simulink model "PMSM_SMO"  (R2023a)
settings: Solver=ode3  StartTime=0.0  StopTime=0.15  FixedStep=2e-7  RelTol=1e-4  EnableMultiTasking=on
InitFcn:
  | R = 0.2875;
  | Ld = 0.002;
  | Lq = 0.004;
  | M=0.4;
  | K=0.2;
values from neighbouring files (symbols this model uses):
  A = [Ld/r Lq/r]    [Motor_PIParam_Get2.m]
  flux = 2.5    [Copy_of_imitate_MPTA_MPTV.m]    (also in Motor_PIParam_Get2.m = 0.646; imitate_MPTA_MPTV.m)
undefined symbols (not defined in the file or in its folder): L
libraries: spsDCVoltageSourceLib x1, spsGroundLib x1, spsPermanentMagnetSynchronousMachineLib x1, simulink x1, spsThreePhaseVIMeasurementLib x1, spsUniversalBridgeLib x1, spspowerguiLib x1
settings Model: Creator=Lei  LastModifiedBy=yll
settings SolverCC: AlgebraicLoopSolver=TrustRegion
settings DataIOCC: LimitDataPoints=on  SaveFormat=Array  SignalLoggingSaveFormat=ModelDataLogs  ReturnWorkspaceOutputs=off
settings OptimizationCC: ExpressionDepthLimit=2147483647  InitFltsAndDblsToZero=on  LifeSpan=inf
settings DebuggingCC: SaveWithParameterizedLinksMsg=none  UnderspecifiedInitializationDetection=Classic  MergeDetectMultiDrivingBlocksExec=none  SignalResolutionControl=TryResolveAllWithWarning  SolverPrmCheckMsg=warning  MultiTaskDSMMsg=warning  MultiTaskCondExecSysMsg=none  FcnCallInpInsideContextMsg=warning  UnconnectedInputMsg=warning  UnconnectedOutputMsg=warning  StateNameClashWarn=warning  SFUnexpectedBacktrackingDiag=warning  SFNoUnconditionalDefaultTransitionDiag=warning  SFExecutionAtInitializationDiag=none  ArithmeticOperatorsInVariantConditions=warning
settings HardwareCC: ProdBitPerPointer=32  ProdBitPerSizeT=32  ProdBitPerPtrDiffT=32  ProdLargestAtomicFloat=None  ProdIntDivRoundTo=Undefined  ProdEndianess=Unspecified  ProdWordSize=32  ProdHWDeviceType=32-bit Generic
settings ModelReferenceCC: PropagateSignalLabelsOutOfModel=off
settings SFSimCC: SimUseLocalCustomCode=off  CustomCodeUndefinedFunction=UseInterfaceOnly
settings RTWCC: RTWUseLocalCustomCode=off
settings CodeAppCC: StateflowObjectComments=on
settings GRTTargetCC: TargetFcnLib=ansi_tfl_tmw.mat  TargetLangStandard=C89/C90 (ANSI)  CombineOutputUpdateFcns=off  GRTInterface=on
settings ConfigComp: CovMetricSettings=dw  CovSaveCumulativeToWorkspaceVar=on  CovSaveSingleToWorkspaceVar=on  CovExternalEMLEnable=off  CovSFcnEnable=off
settings SimscapeCC: SimscapeNormalizeSystem=off

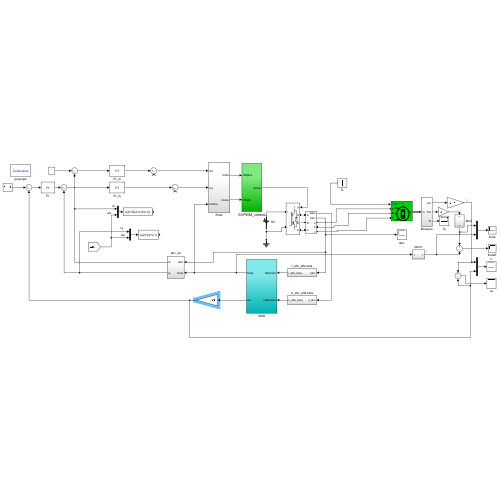
[thumbnail: Simulink's stored preview of the top-level diagram]
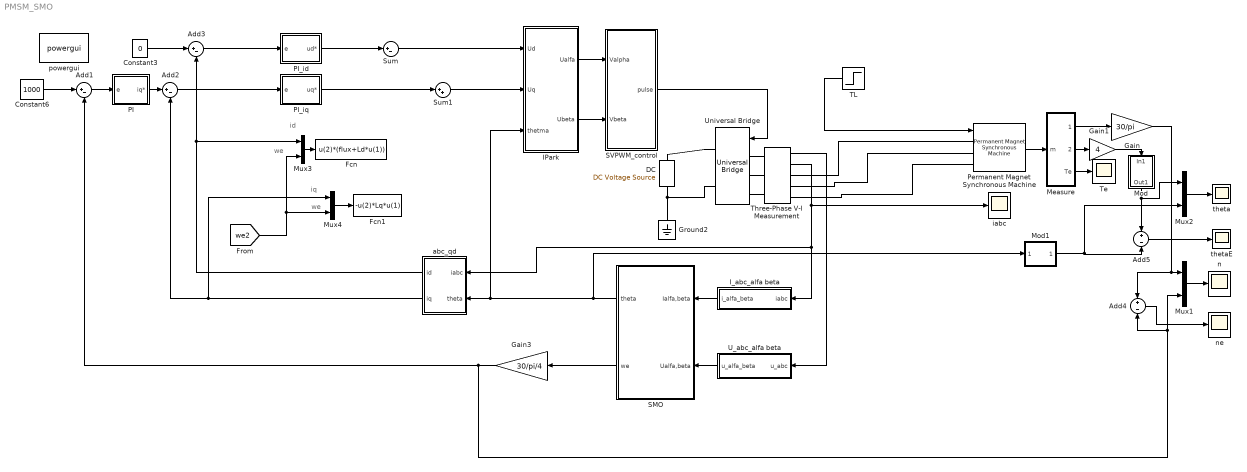
== system PMSM_SMO ==
  note: id
  note: we
  note: iq
  note: we
  Add1 : Sum  Inputs=|+-
  Add2 : Sum  Inputs=|+-
  Add3 : Sum  Inputs=|+-
  Add4 : Sum  Inputs=+|-
  Add5 : Sum  Inputs=+|-
  Constant3 : Constant  Value=0
  Constant6 : Constant  Value=1000
  "DC " : spsDCVoltageSourceLib/DC Voltage Source  Amplitude=311  Measurements=None
  Fcn : Fcn  Expr=u(2)*(flux+Ld*u(1))
  Fcn1 : Fcn  Expr=-u(2)*Lq*u(1)
  Gain : Gain  Gain=30/pi
  Gain1 : Gain  Gain=4
  Gain3 : Gain  Gain=30/pi/4
  Ground2 : spsGroundLib/Ground  LConnTagsString=a
  IPark : Subsystem
  I_abc_alfa beta : Subsystem
  Measure : Subsystem
  Mod : Subsystem
  Mod1 : Subsystem
  Mux{1..4} (4 alike) : Mux  Inputs=2
  PI : Subsystem
      mask Display: disp('PI')
  PI_id : Subsystem
      mask Display: disp('PI')
  PI_iq : Subsystem
      mask Display: disp('PI')
  Permanent Magnet Synchronous Machine : spsPermanentMagnetSynchronousMachineLib/Permanent Magnet Synchronous Machine  NbPhases=3  FluxDistribution=Sinusoidal  RotorType=Salient-pole  MechanicalLoad=Torque Tm  PresetModel=No  ShowDetailedParameters=on  MeasurementBus=off  Resistance=2.8750  Inductance=8.5e-3  dqInductances=[Ld, Lq]  La=0.000835  MachineConstant=Flux linkage established by magnets (V.s)  Flux=0.175  VoltageCst=126.966  TorqueCst=1.05  Flat=120  Mechanical="[ 1e-3, 0,  4 ]"  PolePairs=4  InitialConditions=[0,0, 0,0]  InitialConditions5ph=[0 0 0 0 0 0]  RefAngle=90 degrees behind phase A axis (modified Park)  IterativeDiscreteModel=Trapezoidal non iterative  TsBlock=-1  TsPowergui=0
  SMO : Subsystem
  SVPWM_control : Subsystem
  Sum : Sum  Inputs=|+-
  Sum1 : Sum  Inputs=|++
  TL : Step  Time=0.1  After=0  SampleTime=0
  Te : Scope
  Three-Phase V-I Measurement : spsThreePhaseVIMeasurementLib/Three-Phase V-I Measurement  VoltageMeasurement=phase-to-ground  SetLabelV=off  LabelV=Vabc  Vpu=off  VpuLL=off  CurrentMeasurement=yes  SetLabelI=off  LabelI=Iabc  Ipu=off  Pbase=100e6  Vbase=500e3  OutputType=Complex  PhasorSimulation=off  PSBequivalent=0
  U_abc_alfa beta : Subsystem
  Universal Bridge : spsUniversalBridgeLib/Universal Bridge  Arms=3  SnubberResistance=1e5  SnubberCapacitance=inf  Device=IGBT / Diodes  Ron=1e-3  Lon=0  ForwardVoltages="[  0  0  ]"  ForwardVoltage=0  GTOparameters=[ 10e-6 , 20e-6 ]  IGBTparameters=[ 1e-6 , 2e-6 ]  Measurements=None  Measurements_2=None  converterType=Rectifier
  abc_qd : Subsystem
  iabc : Scope
  n : Scope
  ne : Scope
  powergui : spspowerguiLib/powergui  Priority=1  SimulationMode=Continuous  SampleTime=50e-6  frequency=60  Iterations=50  frequencyindice=0  Pbase=100e6  ErrMax=1e-4  UnitsV=kV  UnitsW=MW  buscounter=0  FunctionMessages=off  echomessages=off  EnableUseOfTLC=off  CurrentSourceSwitches=off  DisableSnubberDevices=off  DisableRonSwitches=off  DisableVfSwitches=off  DisplayEquations=off  AutomaticDiscreteSolvers=off  SolverType=Tustin/Backward Euler (TBE)  Interpol=off  ExternalGateDelay=off  methode=off  Ts=100  x0status=blocks  SPID=off  SwTol=0  HookPort=off  NonlinearTolerance=1e-4  nMaxIteration=100  ContinueOnMaxIteration=off  RestoreLinks=warning  ResistiveCurrentMeasurement=off  Frange=[0:2:500]  Ylog=off  Xlog=on  ShowGrid=off  save=off  variable=ZData  structure=0  ZoomFFT=off  StartTime=0.0  cycles=1  DisplayStyle=1  fundamental=60  FreqAxis=off  MaxFrequency=1000  frequencyindicesteady=1  RmsSteady=1  display=off
  theta : Scope
  thetaE : Scope
  wires:
  Constant3/1 -> Add3/1
  Add1/1 -> PI/1(e)
  Constant6/1 -> Add1/1
  SVPWM_control/1(pulse) -> Universal Bridge/1
  IPark/1(Ualfa) -> SVPWM_control/1(Valpha)
  IPark/2(Ubeta) -> SVPWM_control/2(Vbeta)
  TL/1 -> Permanent Magnet Synchronous Machine/1
  PI/1(iq*) -> Add2/1
  Gain3/1 -> Add1/2, Add4/2, Mux1/2
  SMO/2(we) -> Gain3/1
  Permanent Magnet Synchronous Machine/1 -> Measure/1(m)
  Measure/1(wm) -> Gain/1
  Measure/2(The) -> Gain1/1
  Measure/3(Te) -> Te/1
  Three-Phase V-I Measurement/1 -> U_abc_alfa beta/1(u_abc)
  Add2/1 -> PI_iq/1(e)
  Add3/1 -> PI_id/1(e)
  abc_qd/1(id) -> Mux3/1, Add3/2
  I_abc_alfa beta/1(i_alfa_beta) -> SMO/1(Ialfa,beta)
  U_abc_alfa beta/1(u_alfa_beta) -> SMO/2(Ualfa,beta)
  SMO/1(theta) -> IPark/3(thetma), abc_qd/2(theta), Mod1/1(In1)
  Three-Phase V-I Measurement/2 -> abc_qd/1(iabc), I_abc_alfa beta/1(iabc), iabc/1
  Mux1/1 -> n/1
  Gain/1 -> Add4/1, Mux1/1
  Gain1/1 -> Mod/1(In1)
  Mux2/1 -> theta/1
  Add5/1 -> thetaE/1
  Add4/1 -> ne/1
  Mod/1(Out1) -> Mux2/1, Add5/1
  Mod1/1(Out1) -> Add5/2, Mux2/2
  PI_iq/1(uq*) -> Sum1/1
  Sum1/1 -> IPark/2(Uq)
  Sum/1 -> IPark/1(Ud)
  PI_id/1(ud*) -> Sum/1
  Mux4/1 -> Fcn1/1
  Mux3/1 -> Fcn/1
  abc_qd/2(iq) -> Mux4/1, Add2/2
  [we2] -> Mux4/2, Mux3/2
  connections:
  Universal Bridge/RConn1 -- "DC "/RConn1
  "DC "/LConn1 -- Ground2/LConn1 -- Universal Bridge/RConn2
  Universal Bridge/LConn1 -- Three-Phase V-I Measurement/LConn1
  Universal Bridge/LConn2 -- Three-Phase V-I Measurement/LConn2
  Universal Bridge/LConn3 -- Three-Phase V-I Measurement/LConn3
  Three-Phase V-I Measurement/RConn1 -- Permanent Magnet Synchronous Machine/LConn1
  Three-Phase V-I Measurement/RConn2 -- Permanent Magnet Synchronous Machine/LConn2
  Three-Phase V-I Measurement/RConn3 -- Permanent Magnet Synchronous Machine/LConn3

== system PMSM_SMO/IPark ==
  Ud : Inport
  Uq : Inport  Port=2
  thetma : Inport  Port=3
  Fcn : Fcn  Expr=cos(u[3])*u[2]-sin(u[3])*u[1]
  Fcn1 : Fcn  Expr=sin(u[3])*u[2]+cos(u[3])*u[1]
  Mux : Mux  Inputs=3
  Ualfa : Outport
  Ubeta : Outport  Port=2
  wires:
  Uq/1 -> Mux/1
  Ud/1 -> Mux/2
  thetma/1 -> Mux/3
  Mux/1 -> Fcn/1, Fcn1/1
  Fcn/1 -> Ualfa/1
  Fcn1/1 -> Ubeta/1

== system PMSM_SMO/I_abc_alfa beta ==
  iabc : Inport
  Fcn : Fcn  Expr=(2*u(1)-u(2)-u(3))/3
  Fcn1 : Fcn  Expr=(u(2)-u(3))/(3^(1/2))
  Mux2 : Mux  Inputs=2
  i_alfa_beta : Outport
  wires:
  iabc/1 -> Fcn/1, Fcn1/1
  Mux2/1 -> i_alfa_beta/1
  Fcn/1 -> Mux2/1
  Fcn1/1 -> Mux2/2

== system PMSM_SMO/Measure ==
  m : Inport
  Bus Selector1 : BusSelector  OutputSignals=Rotor speed wm (rad/s),Rotor angle thetam (rad),Electromagnetic torque Te (N*m)
  wm : Outport
  The : Outport  Port=2
  Te : Outport  Port=3
  wires:
  Bus Selector1/2 -> The/1  "<Rotor angle thetam (rad)>"
  Bus Selector1/3 -> Te/1  "<Electromagnetic torque Te (N*m)>"
  m/1 -> Bus Selector1/1
  Bus Selector1/1 -> wm/1  "<Rotor speed wm (rad/s)>"

== system PMSM_SMO/Mod ==
  In1 : Inport
  Constant1 : Constant  Value=pi/4
  Math Function : Math  Operator=mod  SignedPower=on
  Out1 : Outport
  wires:
  Constant1/1 -> Math Function/2
  Math Function/1 -> Out1/1
  In1/1 -> Math Function/1

== system PMSM_SMO/Mod1 ==
  In1 : Inport
  Constant1 : Constant  Value=pi/4
  Math Function : Math  Operator=mod  SignedPower=on
  Out1 : Outport
  wires:
  In1/1 -> Math Function/1
  Math Function/1 -> Out1/1
  Constant1/1 -> Math Function/2

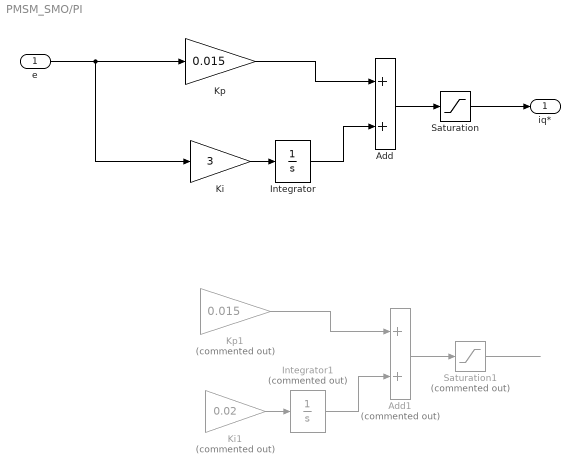
== system PMSM_SMO/PI ==
  e : Inport
  Add : Sum
  Add1 : Sum  Commented=on
  Integrator : Integrator
  Integrator1 : Integrator  Commented=on
  Ki : Gain  Gain=3
  Ki1 : Gain  Commented=on  Gain=0.02
  Kp : Gain  Gain=0.015
  Kp1 : Gain  Commented=on  Gain=0.015
  Saturation : Saturate  UpperLimit=21  LowerLimit=-21
  Saturation1 : Saturate  Commented=on  UpperLimit=21  LowerLimit=-21
  iq* : Outport
  wires:
  Saturation/1 -> iq*/1
  Ki/1 -> Integrator/1
  e/1 -> Kp/1, Ki/1
  Integrator/1 -> Add/2
  Kp/1 -> Add/1
  Add/1 -> Saturation/1
  Kp1/1 -> Add1/1
  Integrator1/1 -> Add1/2
  Ki1/1 -> Integrator1/1
  ? -> Kp1/1, Ki1/1
  Add1/1 -> Saturation1/1
  Saturation1/1 -> ?

== system PMSM_SMO/PI_id ==
  e : Inport
  Add : Sum
  Integrator : Integrator
  Integrator1 : Integrator
  Ki : Gain  Gain=R*2000
  Ki1 : Gain  Gain=R*2000
  Kp : Gain  Gain=20
  Kp1 : Gain  Gain=20
  Saturation : Saturate  UpperLimit=350  LowerLimit=-350
  ud* : Outport
  wires:
  Ki/1 -> Integrator/1
  e/1 -> Kp/1, Ki/1
  Saturation/1 -> ud*/1
  Integrator/1 -> Add/2
  Kp/1 -> Add/1
  Add/1 -> Saturation/1
  Integrator1/1 -> ?
  ? -> Ki1/1
  ? -> Kp1/1
  Kp1/1 -> ?
  Ki1/1 -> Integrator1/1

== system PMSM_SMO/PI_iq ==
  e : Inport
  Add : Sum
  Integrator : Integrator
  Ki : Gain  Gain=R*2000
  Kp : Gain  Gain=20
  Saturation : Saturate  UpperLimit=350  LowerLimit=-350
  uq* : Outport
  wires:
  Ki/1 -> Integrator/1
  e/1 -> Kp/1, Ki/1
  Saturation/1 -> uq*/1
  Integrator/1 -> Add/2
  Kp/1 -> Add/1
  Add/1 -> Saturation/1

== system PMSM_SMO/SMO ==
  Ialfa,beta : Inport
  Ualfa,beta : Inport  Port=2
  Arctan_function1 : Subsystem
  FULL_SMO : Subsystem
  PLL : Subsystem
  SMO : Subsystem
  theta : Outport
  we : Outport  Port=2
  tag scope: we2=global
  wires:
  Arctan_function1/1(theta) -> theta/1
  Arctan_function1/2(we) -> [we2], we/1
  Ualfa,beta/1 -> FULL_SMO/1(Ualfa,beta)
  Ialfa,beta/1 -> FULL_SMO/2(Ialfa,beta)
  FULL_SMO/1(Ealpha^) -> Arctan_function1/1(Ealpha^)
  FULL_SMO/2(Ebeta^) -> Arctan_function1/2(Ebeta)

== system PMSM_SMO/SVPWM_control ==
  Valpha : Inport
  Vbeta : Inport  Port=2
  Repeating Sequence : simulink/Sources/Repeating Sequence  rep_seq_t=[0 0.0001 0.0002]  rep_seq_y=[0 0.0001 0]
  Subsystem : Subsystem
  Subsystem1 : Subsystem
  Subsystem2 : Subsystem
  Subsystem3 : Subsystem
  Subsystem4 : Subsystem
  Subsystem5 : Subsystem
  T : Constant  Value=0.0001
  Vdc : Constant  Value=311
  pulse : Outport
  wires:
  Subsystem5/1(g) -> pulse/1
  Repeating Sequence/1 -> Subsystem5/1(In1)
  Subsystem4/3(Tcm3) -> Subsystem5/4(In4)
  Subsystem4/2(Tcm2) -> Subsystem5/3(In3)
  Subsystem4/1(Tcm1) -> Subsystem5/2(In2)
  Subsystem3/3(Tc) -> Subsystem4/4(In4)
  Subsystem3/2(Tb) -> Subsystem4/3(In3)
  Subsystem3/1(Ta) -> Subsystem4/2(In2)
  Subsystem2/2(T2) -> Subsystem3/3(T2)
  Subsystem2/1(T1) -> Subsystem3/1(T1)
  Subsystem1/3(Z) -> Subsystem2/4(In4)
  Subsystem1/2(Y) -> Subsystem2/3(In3)
  Subsystem1/1(x) -> Subsystem2/2(In2)
  Subsystem/1(N) -> Subsystem4/1(In1), Subsystem2/1(In1)
  Vdc/1 -> Subsystem1/4(Vdc)
  T/1 -> Subsystem3/2(T), Subsystem1/1(T)
  Vbeta/1 -> Subsystem1/2(In2), Subsystem/2(Vbeta)
  Valpha/1 -> Subsystem1/3(In3), Subsystem/1(Valpha)

== system PMSM_SMO/U_abc_alfa beta ==
  u_abc : Inport
  Fcn : Fcn  Expr=(2*u(1)-u(2)-u(3))/3
  Fcn1 : Fcn  Expr=(u(2)-u(3))/(3^(1/2))
  Mux2 : Mux  Inputs=2
  u_alfa_beta : Outport
  wires:
  u_abc/1 -> Fcn/1, Fcn1/1
  Mux2/1 -> u_alfa_beta/1
  Fcn/1 -> Mux2/1
  Fcn1/1 -> Mux2/2

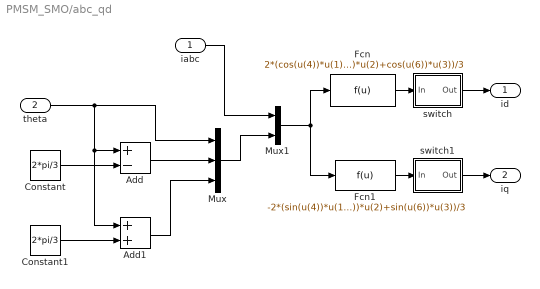
== system PMSM_SMO/abc_qd ==
  iabc : Inport
  theta : Inport  Port=2
  Add : Sum  Inputs=+-
  Add1 : Sum
  Constant : Constant  Value=2*pi/3
  Constant1 : Constant  Value=2*pi/3
  Fcn : Fcn  Expr=2*(cos(u(4))*u(1)+cos(u(5))*u(2)+cos(u(6))*u(3))/3
  Fcn1 : Fcn  Expr=-2*(sin(u(4))*u(1)+sin(u(5))*u(2)+sin(u(6))*u(3))/3
  Mux : Mux  Inputs=3
  Mux1 : Mux  Inputs=2
  switch : Subsystem
  switch1 : Subsystem
  id : Outport
  iq : Outport  Port=2
  wires:
  Constant1/1 -> Add1/2
  Constant/1 -> Add/2
  theta/1 -> Mux/1, Add1/1, Add/1
  Add/1 -> Mux/2
  Add1/1 -> Mux/3
  Mux/1 -> Mux1/2
  iabc/1 -> Mux1/1
  Mux1/1 -> Fcn/1, Fcn1/1
  Fcn/1 -> switch/1(In)
  switch/1(Out) -> id/1
  Fcn1/1 -> switch1/1(In)
  switch1/1(Out) -> iq/1

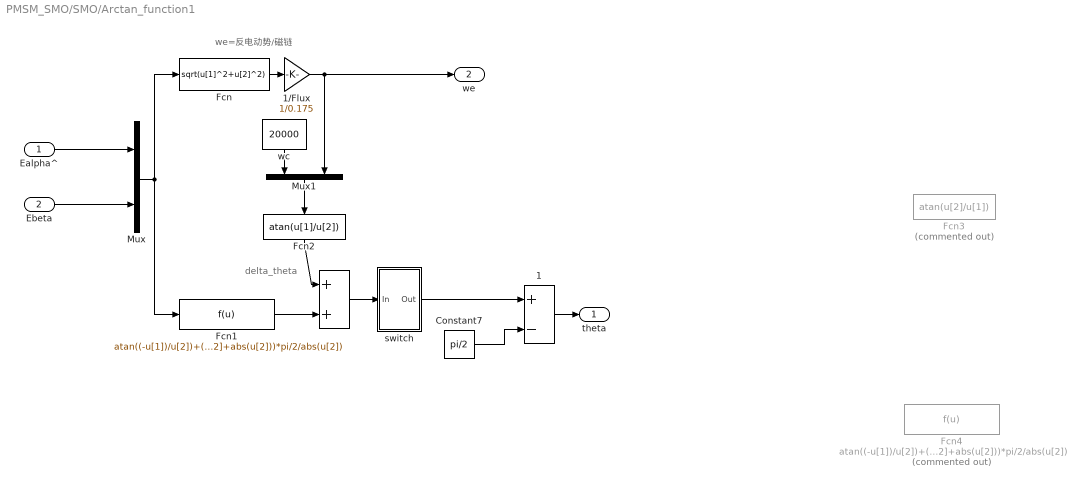
== system PMSM_SMO/SMO/Arctan_function1 ==
  note: we=反电动势/磁链
  note: delta_theta
  Ealpha^ : Inport
  Ebeta : Inport  Port=2
  "  " : Sum
  "  1" : Sum  Inputs=+-
  1/Flux : Gain  Gain=1/0.175
  Constant7 : Constant  Value=pi/2
  Fcn : Fcn  Expr=sqrt(u[1]^2+u[2]^2)
  Fcn1 : Fcn  Expr=atan((-u[1])/u[2])+(-u[2]+abs(u[2]))*pi/2/abs(u[2])
  Fcn2 : Fcn  Expr=atan(u[1]/u[2])
  Fcn3 : Fcn  Commented=on  Expr=atan(u[2]/u[1])
  Fcn4 : Fcn  Commented=on  Expr=atan((-u[1])/u[2])+(-u[2]+abs(u[2]))*pi/2/abs(u[2])
  Mux : Mux  Inputs=2
  Mux1 : Mux  Inputs=2
  switch : Subsystem
  wc : Constant  Value=20000
  theta : Outport
  we : Outport  Port=2
  wires:
  Mux/1 -> Fcn/1, Fcn1/1
  Fcn/1 -> 1/Flux/1
  1/Flux/1 -> we/1, Mux1/2
  Fcn1/1 -> "  "/2
  "  "/1 -> switch/1(In)
  Mux1/1 -> Fcn2/1
  Fcn2/1 -> "  "/1
  wc/1 -> Mux1/1
  switch/1(Out) -> "  1"/1
  Ebeta/1 -> Mux/2
  Ealpha^/1 -> Mux/1
  Constant7/1 -> "  1"/2
  "  1"/1 -> theta/1

== system PMSM_SMO/SMO/FULL_SMO ==
  note: 低通滤波器
  Ualfa,beta : Inport
  Ialfa,beta : Inport  Port=2
  Demux1 : Demux  Outputs=2
  Demux2 : Demux  Outputs=2
  凸极 : Subsystem
  Ealpha^ : Outport
  Ebeta^ : Outport  Port=2
  wires:
  Demux2/2 -> 凸极/4(Ibeta)
  Demux2/1 -> 凸极/3(Ialfa)
  Demux1/2 -> 凸极/2(Ubeta)
  Demux1/1 -> 凸极/1(Ualfa)
  Ualfa,beta/1 -> Demux1/1
  Ialfa,beta/1 -> Demux2/1
  凸极/1(E_alpha_pre) -> Ealpha^/1
  凸极/2(E_beta_pre) -> Ebeta^/1

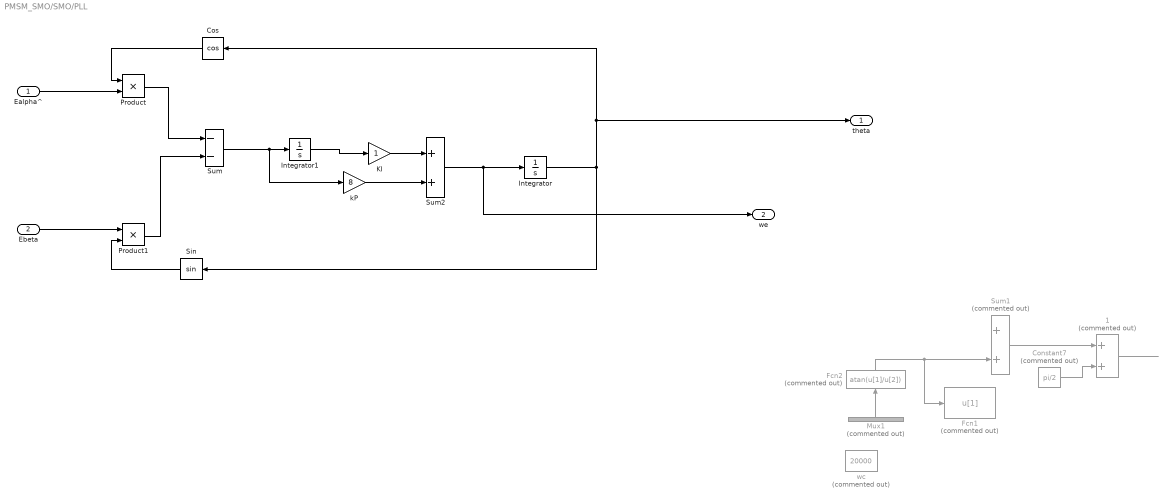
== system PMSM_SMO/SMO/PLL ==
  Ealpha^ : Inport
  Ebeta : Inport  Port=2
  "  1" : Sum  Commented=on
  Constant7 : Constant  Commented=on  Value=pi/2
  Cos : Trigonometry  Operator=cos
  Fcn1 : Fcn  Commented=on  Expr=u[1]
  Fcn2 : Fcn  Commented=on  Expr=atan(u[1]/u[2])
  Integrator : Integrator
  Integrator1 : Integrator
  KI : Gain
  Mux1 : Mux  Commented=on  Inputs=2
  Product : Product
  Product1 : Product
  Sin : Trigonometry
  Sum : Sum  Inputs=--
  Sum1 : Sum  Commented=on
  Sum2 : Sum
  kP : Gain  Gain=8
  wc : Constant  Commented=on  Value=20000
  theta : Outport
  we : Outport  Port=2
  wires:
  Product/1 -> Sum/1
  Product1/1 -> Sum/2
  Cos/1 -> Product/1
  Sin/1 -> Product1/2
  kP/1 -> Sum2/2
  KI/1 -> Sum2/1
  Integrator1/1 -> KI/1
  Sum/1 -> kP/1, Integrator1/1
  Ebeta/1 -> Product1/1
  Ealpha^/1 -> Product/2
  Sum1/1 -> "  1"/1
  Constant7/1 -> "  1"/2
  "  1"/1 -> ?
  Fcn2/1 -> Fcn1/1, Sum1/2
  ? -> Mux1/2
  ? -> Sum1/1
  Mux1/1 -> Fcn2/1
  Sum2/1 -> we/1, Integrator/1
  Integrator/1 -> Cos/1, theta/1, Sin/1

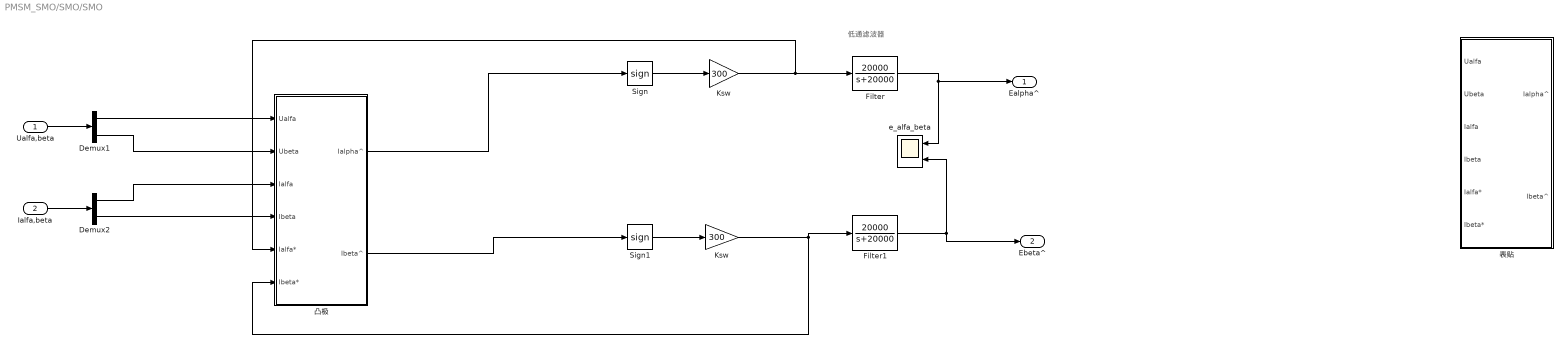
== system PMSM_SMO/SMO/SMO ==
  note: 低通滤波器
  Ualfa,beta : Inport
  Ialfa,beta : Inport  Port=2
  Demux1 : Demux  Outputs=2
  Demux2 : Demux  Outputs=2
  Filter : TransferFcn  Numerator=[20000]  Denominator=[1 20000]
  Filter1 : TransferFcn  Numerator=[20000]  Denominator=[1 20000]
  Ksw : Gain  Gain=300
  "Ksw " : Gain  Gain=300
  Sign : Signum  ZeroCross=off
  Sign1 : Signum  ZeroCross=off
  e_alfa_beta : Scope  NumInputPorts=2
  凸极 : Subsystem
  表贴 : Subsystem
  Ealpha^ : Outport
  Ebeta^ : Outport  Port=2
  wires:
  Sign/1 -> Ksw/1
  Ksw/1 -> 凸极/5(Ialfa*), Filter/1
  Sign1/1 -> "Ksw "/1
  "Ksw "/1 -> 凸极/6(Ibeta*), Filter1/1
  Filter1/1 -> Ebeta^/1, e_alfa_beta/2
  Filter/1 -> Ealpha^/1, e_alfa_beta/1
  Ialfa,beta/1 -> Demux2/1
  Ualfa,beta/1 -> Demux1/1
  Demux1/1 -> 凸极/1(Ualfa)
  Demux1/2 -> 凸极/2(Ubeta)
  Demux2/1 -> 凸极/3(Ialfa)
  Demux2/2 -> 凸极/4(Ibeta)
  凸极/1(Ialpha^) -> Sign/1
  凸极/2(Ibeta^) -> Sign1/1

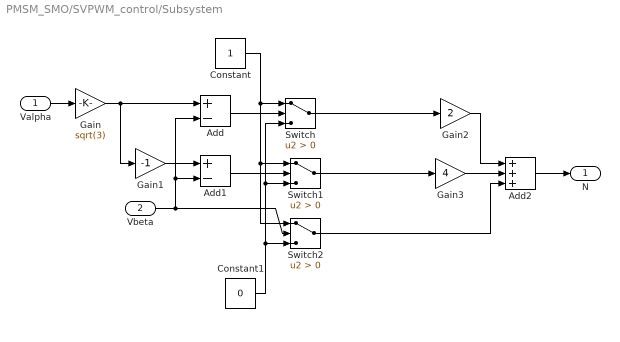
== system PMSM_SMO/SVPWM_control/Subsystem ==
  Valpha : Inport
  Vbeta : Inport  Port=2
  Add : Sum  Inputs=+-
  Add1 : Sum  Inputs=+-
  Add2 : Sum  Inputs=+++
  Constant : Constant
  Constant1 : Constant  Value=0
  Gain : Gain  Gain=sqrt(3)
  Gain1 : Gain  Gain=-1
  Gain2 : Gain  Gain=2
  Gain3 : Gain  Gain=4
  Switch : Switch  Criteria=u2 > Threshold  SaturateOnIntegerOverflow=off  InputSameDT=off
  Switch1 : Switch  Criteria=u2 > Threshold  SaturateOnIntegerOverflow=off  InputSameDT=off
  Switch2 : Switch  Criteria=u2 > Threshold  SaturateOnIntegerOverflow=off  InputSameDT=off
  N : Outport
  wires:
  Valpha/1 -> Gain/1
  Gain3/1 -> Add2/2
  Gain2/1 -> Add2/1
  Add1/1 -> Switch1/2
  Gain1/1 -> Add1/1
  Switch1/1 -> Gain3/1
  Switch2/1 -> Add2/3
  Switch/1 -> Gain2/1
  Add/1 -> Switch/2
  Gain/1 -> Gain1/1, Add/1
  Constant1/1 -> Switch/3, Switch1/3, Switch2/3
  Constant/1 -> Switch1/1, Switch2/1, Switch/1
  Vbeta/1 -> Add1/2, Add/2, Switch2/2
  Add2/1 -> N/1

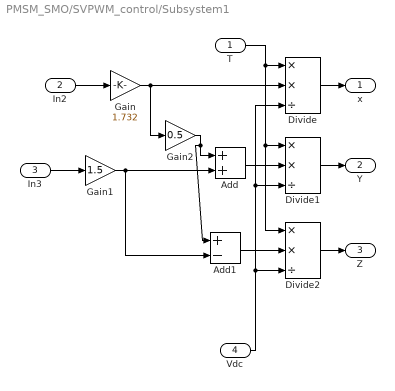
== system PMSM_SMO/SVPWM_control/Subsystem1 ==
  T : Inport
  In2 : Inport  Port=2
  In3 : Inport  Port=3
  Vdc : Inport  Port=4
  Add : Sum
  Add1 : Sum  Inputs=+-
  Divide : Product  Inputs=**/
  Divide1 : Product  Inputs=**/
  Divide2 : Product  Inputs=**/
  Gain : Gain  Gain=1.732
  Gain1 : Gain  Gain=1.5
  Gain2 : Gain  Gain=0.5
  x : Outport
  Y : Outport  Port=2
  Z : Outport  Port=3
  wires:
  Divide2/1 -> Z/1
  Divide1/1 -> Y/1
  Divide/1 -> x/1
  In3/1 -> Gain1/1
  In2/1 -> Gain/1
  Add1/1 -> Divide2/2
  Add/1 -> Divide1/2
  Gain1/1 -> Add1/2, Add/2
  Gain2/1 -> Add1/1, Add/1
  Gain/1 -> Gain2/1, Divide/2
  Vdc/1 -> Divide/3, Divide1/3, Divide2/3
  T/1 -> Divide2/1, Divide1/1, Divide/1

== system PMSM_SMO/SVPWM_control/Subsystem2 ==
  In1 : Inport
  In2 : Inport  Port=2
  In3 : Inport  Port=3
  In4 : Inport  Port=4
  Gain : Gain  Gain=-1
  Gain1 : Gain  Gain=-1
  Gain2 : Gain  Gain=-1
  Multiport Switch : MultiPortSwitch  Inputs=6  SaturateOnIntegerOverflow=off  InputSameDT=off
  Multiport Switch1 : MultiPortSwitch  Inputs=6  SaturateOnIntegerOverflow=off  InputSameDT=off
  T1 : Outport
  T2 : Outport  Port=2
  wires:
  Multiport Switch1/1 -> T2/1
  Multiport Switch/1 -> T1/1
  Gain2/1 -> Multiport Switch/7, Multiport Switch1/6
  Gain1/1 -> Multiport Switch1/3, Multiport Switch/5
  In2/1 -> Gain1/1, Multiport Switch/6, Multiport Switch1/4
  Gain/1 -> Multiport Switch1/7, Multiport Switch/4
  In3/1 -> Gain2/1, Multiport Switch1/2, Multiport Switch/3
  In4/1 -> Gain/1, Multiport Switch/2, Multiport Switch1/5
  In1/1 -> Multiport Switch/1, Multiport Switch1/1

== system PMSM_SMO/SVPWM_control/Subsystem3 ==
  T1 : Inport
  T : Inport  Port=2
  T2 : Inport  Port=3
  Add : Sum  Inputs=--+
  Add1 : Sum
  Add2 : Sum
  Gain : Gain  Gain=0.25
  Gain1 : Gain  Gain=0.5
  Gain2 : Gain  Gain=0.5
  Ta : Outport
  Tb : Outport  Port=2
  Tc : Outport  Port=3
  wires:
  T/1 -> Add/3
  Add2/1 -> Tc/1
  Gain2/1 -> Add2/2
  Add1/1 -> Add2/1, Tb/1
  Gain1/1 -> Add1/2
  Gain/1 -> Add1/1, Ta/1
  Add/1 -> Gain/1
  T2/1 -> Add/2, Gain2/1
  T1/1 -> Add/1, Gain1/1

== system PMSM_SMO/SVPWM_control/Subsystem4 ==
  In1 : Inport
  In2 : Inport  Port=2
  In3 : Inport  Port=3
  In4 : Inport  Port=4
  Multiport Switch : MultiPortSwitch  Inputs=6  SaturateOnIntegerOverflow=off  InputSameDT=off
  Multiport Switch1 : MultiPortSwitch  Inputs=6  SaturateOnIntegerOverflow=off  InputSameDT=off
  Multiport Switch2 : MultiPortSwitch  Inputs=6  SaturateOnIntegerOverflow=off  InputSameDT=off
  Tcm1 : Outport
  Tcm2 : Outport  Port=2
  Tcm3 : Outport  Port=3
  wires:
  Multiport Switch2/1 -> Tcm3/1
  Multiport Switch1/1 -> Tcm2/1
  Multiport Switch/1 -> Tcm1/1
  In1/1 -> Multiport Switch2/1, Multiport Switch1/1, Multiport Switch/1
  In4/1 -> Multiport Switch1/3, Multiport Switch1/7, Multiport Switch2/2, Multiport Switch2/4, Multiport Switch/5, Multiport Switch/6
  In2/1 -> Multiport Switch/4, Multiport Switch/3, Multiport Switch1/2, Multiport Switch1/6, Multiport Switch2/5, Multiport Switch2/7
  In3/1 -> Multiport Switch/2, Multiport Switch/7, Multiport Switch1/4, Multiport Switch1/5, Multiport Switch2/3, Multiport Switch2/6

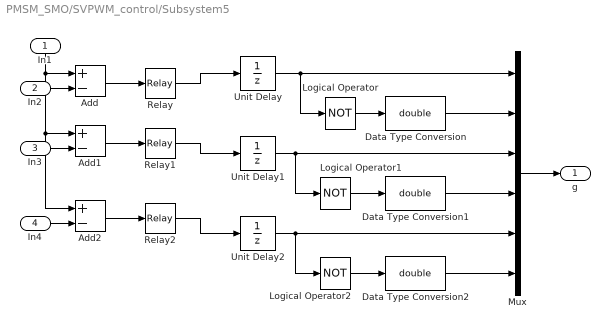
== system PMSM_SMO/SVPWM_control/Subsystem5 ==
  In1 : Inport
  In2 : Inport  Port=2
  In3 : Inport  Port=3
  In4 : Inport  Port=4
  Add : Sum  Inputs=+-
  Add1 : Sum  Inputs=+-
  Add2 : Sum  Inputs=+-
  Data Type Conversion : DataTypeConversion  OutDataTypeStr=double  SaturateOnIntegerOverflow=off  RndMeth=Floor
  Data Type Conversion1 : DataTypeConversion  OutDataTypeStr=double  SaturateOnIntegerOverflow=off  RndMeth=Floor
  Data Type Conversion2 : DataTypeConversion  OutDataTypeStr=double  SaturateOnIntegerOverflow=off  RndMeth=Floor
  Logical Operator : Logic  Operator=NOT  AllPortsSameDT=off  OutDataTypeStr=boolean
  Logical Operator1 : Logic  Operator=NOT  AllPortsSameDT=off  OutDataTypeStr=boolean
  Logical Operator2 : Logic  Operator=NOT  AllPortsSameDT=off  OutDataTypeStr=boolean
  Mux : Mux  Inputs=6
  Relay : Relay  OffSwitchValue=-eps
  Relay1 : Relay  OffSwitchValue=-eps
  Relay2 : Relay  OffSwitchValue=-eps
  Unit Delay : UnitDelay  SampleTime=-1  HasFrameUpgradeWarning=on
  Unit Delay1 : UnitDelay  SampleTime=-1  HasFrameUpgradeWarning=on
  Unit Delay2 : UnitDelay  SampleTime=-1  HasFrameUpgradeWarning=on
  g : Outport
  wires:
  In4/1 -> Add2/2
  In3/1 -> Add1/2
  In2/1 -> Add/2
  Relay2/1 -> Unit Delay2/1
  Relay1/1 -> Unit Delay1/1
  Relay/1 -> Unit Delay/1
  Unit Delay2/1 -> Mux/5, Logical Operator2/1
  Unit Delay1/1 -> Mux/3, Logical Operator1/1
  Unit Delay/1 -> Logical Operator/1, Mux/1
  Mux/1 -> g/1
  Data Type Conversion/1 -> Mux/2
  Data Type Conversion1/1 -> Mux/4
  Data Type Conversion2/1 -> Mux/6
  Logical Operator2/1 -> Data Type Conversion2/1
  Logical Operator1/1 -> Data Type Conversion1/1
  Logical Operator/1 -> Data Type Conversion/1
  Add1/1 -> Relay1/1
  Add2/1 -> Relay2/1
  Add/1 -> Relay/1
  In1/1 -> Add/1, Add2/1, Add1/1

== system PMSM_SMO/abc_qd/switch ==
  In : Inport
  Constant4 : Constant  Value=0
  Step1 : Step  Time=0.001  SampleTime=0
  Switch : Switch  Threshold=1  SaturateOnIntegerOverflow=off  InputSameDT=off
  Out : Outport
  wires:
  Step1/1 -> Switch/2
  Constant4/1 -> Switch/3
  In/1 -> Switch/1
  Switch/1 -> Out/1

== system PMSM_SMO/abc_qd/switch1 ==
  In : Inport
  Constant4 : Constant  Value=0
  Step1 : Step  Time=0.001  SampleTime=0
  Switch : Switch  Threshold=1  SaturateOnIntegerOverflow=off  InputSameDT=off
  Out : Outport
  wires:
  Switch/1 -> Out/1
  In/1 -> Switch/1
  Constant4/1 -> Switch/3
  Step1/1 -> Switch/2

== system PMSM_SMO/SMO/Arctan_function1/switch ==
  In : Inport
  Constant4 : Constant  Value=0
  Step1 : Step  Time=0.001  SampleTime=0
  Switch : Switch  Threshold=1  SaturateOnIntegerOverflow=off  InputSameDT=off
  Out : Outport
  wires:
  Step1/1 -> Switch/2
  Constant4/1 -> Switch/3
  In/1 -> Switch/1
  Switch/1 -> Out/1

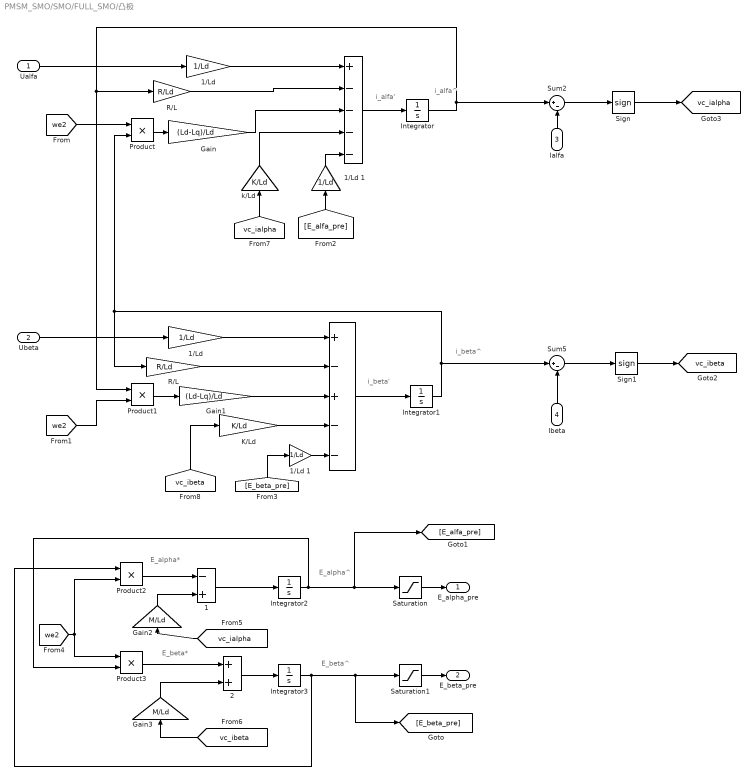
== system PMSM_SMO/SMO/FULL_SMO/凸极 ==
  note: E_beta^
  note: i_beta^
  note: i_alfa'
  note: i_beta'
  note: i_alfa^
  note: E_alpha^
  note: E_beta*
  note: E_alpha*
  Ualfa : Inport
  Ubeta : Inport  Port=2
  Ialfa : Inport  Port=3
  Ibeta : Inport  Port=4
  " " : Sum  Inputs=+----
  "   " : Sum  Inputs=+-+--
  "   1" : Sum  Inputs=-+
  "   2" : Sum
  " 1/Ld" : Gain  Gain=1/Ld
  " 1/Ld 1" : Gain  Gain=1/Ld
  1/Ld : Gain  Gain=1/Ld
  1/Ld 1 : Gain  Gain=1/Ld
  Gain : Gain  Gain=(Ld-Lq)/Ld
  Gain1 : Gain  Gain=(Ld-Lq)/Ld
  Gain2 : Gain  Gain=M/Ld
  Gain3 : Gain  Gain=M/Ld
  Integrator{,1..3} (4 alike) : Integrator
  K/Ld : Gain  Gain=K/Ld
  Product{,1..3} (4 alike) : Product
  R/L : Gain  Gain=R/Ld
  "R/L " : Gain  Gain=R/Ld
  Saturation : Saturate  UpperLimit=3000  LowerLimit=-3000
  Saturation1 : Saturate  UpperLimit=3000  LowerLimit=-3000
  Sign : Signum  ZeroCross=off
  Sign1 : Signum  ZeroCross=off
  Sum2 : Sum  Inputs=|+-
  Sum5 : Sum  Inputs=|+-
  "k/Ld " : Gain  Gain=K/Ld
  E_alpha_pre : Outport
  E_beta_pre : Outport  Port=2
  tag scope: vc_ialpha=global, vc_ibeta=global
  wires:
  [we2] -> Product1/2
  Gain1/1 -> "   "/3
  Product1/1 -> Gain1/1
  Gain/1 -> " "/3
  Product/1 -> Gain/1
  [we2] -> Product/1
  Ialfa/1 -> Sum2/2
  Ibeta/1 -> Sum5/2
  Integrator1/1 -> Product/2, "R/L "/1, Sum5/1
  Ubeta/1 -> " 1/Ld"/1
  1/Ld/1 -> " "/1
  " 1/Ld"/1 -> "   "/1
  " "/1 -> Integrator/1
  Ualfa/1 -> 1/Ld/1
  K/Ld/1 -> "   "/4
  Integrator/1 -> R/L/1, Product1/1, Sum2/1
  "R/L "/1 -> "   "/2
  "k/Ld "/1 -> " "/4
  "   "/1 -> Integrator1/1
  R/L/1 -> " "/2
  1/Ld 1/1 -> " "/5
  [E_alfa_pre] -> 1/Ld 1/1
  " 1/Ld 1"/1 -> "   "/5
  [E_beta_pre] -> " 1/Ld 1"/1
  [we2] -> Product2/2, Product3/1
  Integrator2/1 -> [E_alfa_pre], Saturation/1, Product3/2
  "   1"/1 -> Integrator2/1
  Product2/1 -> "   1"/1
  "   2"/1 -> Integrator3/1
  Product3/1 -> "   2"/1
  [vc_ibeta] -> Gain3/1
  Gain3/1 -> "   2"/2
  [vc_ialpha] -> Gain2/1
  Integrator3/1 -> [E_beta_pre], Saturation1/1, Product2/1
  Sum2/1 -> Sign/1
  Sum5/1 -> Sign1/1
  Sign1/1 -> [vc_ibeta]
  Sign/1 -> [vc_ialpha]
  [vc_ialpha] -> "k/Ld "/1
  [vc_ibeta] -> K/Ld/1
  Gain2/1 -> "   1"/2
  Saturation1/1 -> E_beta_pre/1
  Saturation/1 -> E_alpha_pre/1

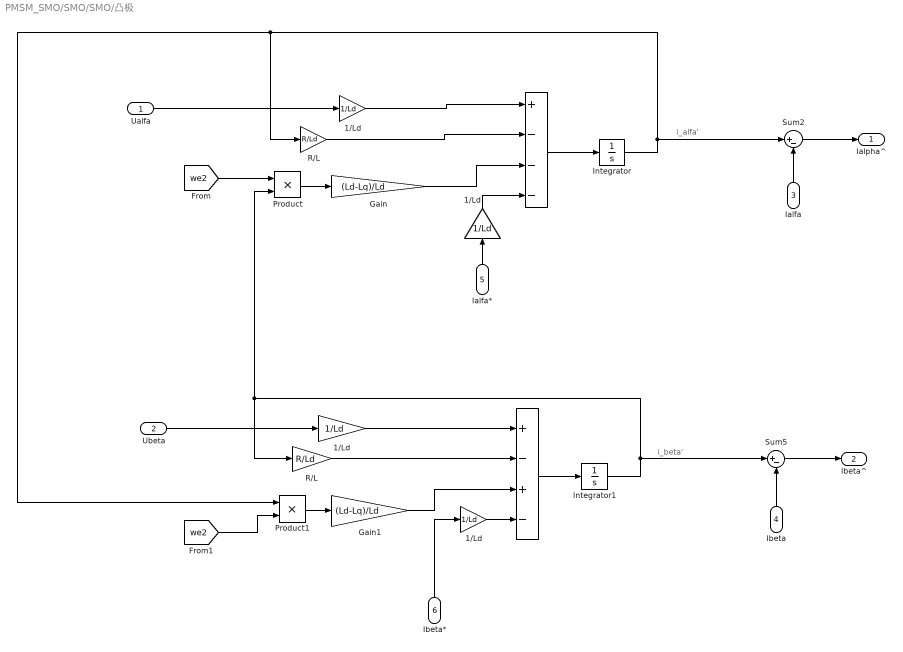
== system PMSM_SMO/SMO/SMO/凸极 ==
  note: i_beta'
  note: i_alfa'
  Ualfa : Inport
  Ubeta : Inport  Port=2
  Ialfa : Inport  Port=3
  Ibeta : Inport  Port=4
  Ialfa* : Inport  Port=5
  Ibeta* : Inport  Port=6
  " " : Sum  Inputs=+---
  "   " : Sum  Inputs=+-+-
  " 1/Ld" : Gain  Gain=1/Ld
  " 1/Ld " : Gain  Gain=1/Ld
  1/Ld : Gain  Gain=1/Ld
  "1/Ld " : Gain  Gain=1/Ld
  Gain : Gain  Gain=(Ld-Lq)/Ld
  Gain1 : Gain  Gain=(Ld-Lq)/Ld
  Integrator : Integrator
  Integrator1 : Integrator
  Product : Product
  Product1 : Product
  R/L : Gain  Gain=R/Ld
  "R/L " : Gain  Gain=R/Ld
  Sum2 : Sum  Inputs=|+-
  Sum5 : Sum  Inputs=|+-
  Ialpha^ : Outport
  Ibeta^ : Outport  Port=2
  wires:
  R/L/1 -> " "/2
  "   "/1 -> Integrator1/1
  "1/Ld "/1 -> " "/4
  "R/L "/1 -> "   "/2
  Integrator/1 -> Sum2/1, R/L/1, Product1/1
  " 1/Ld "/1 -> "   "/4
  Ualfa/1 -> 1/Ld/1
  " "/1 -> Integrator/1
  " 1/Ld"/1 -> "   "/1
  Sum2/1 -> Ialpha^/1
  1/Ld/1 -> " "/1
  Ubeta/1 -> " 1/Ld"/1
  Integrator1/1 -> Sum5/1, "R/L "/1, Product/2
  Sum5/1 -> Ibeta^/1
  Ibeta/1 -> Sum5/2
  Ialfa/1 -> Sum2/2
  Ialfa*/1 -> "1/Ld "/1
  Ibeta*/1 -> " 1/Ld "/1
  [we2] -> Product/1
  Product/1 -> Gain/1
  Gain/1 -> " "/3
  Product1/1 -> Gain1/1
  Gain1/1 -> "   "/3
  [we2] -> Product1/2

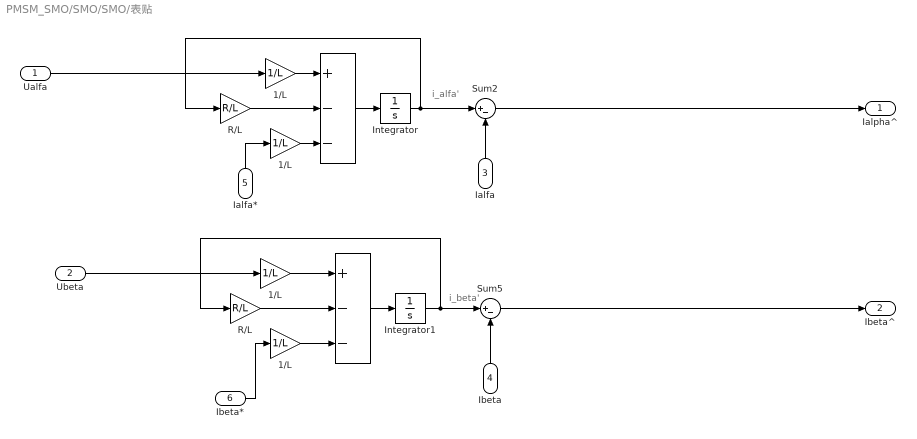
== system PMSM_SMO/SMO/SMO/表贴 ==
  note: i_alfa'
  note: i_beta'
  Ualfa : Inport
  Ubeta : Inport  Port=2
  Ialfa : Inport  Port=3
  Ibeta : Inport  Port=4
  Ialfa* : Inport  Port=5
  Ibeta* : Inport  Port=6
  " " : Sum  Inputs=+--
  "   " : Sum  Inputs=+--
  " 1/L" : Gain  Gain=1/L
  " 1/L " : Gain  Gain=1/L
  1/L : Gain  Gain=1/L
  "1/L " : Gain  Gain=1/L
  Integrator : Integrator
  Integrator1 : Integrator
  R/L : Gain  Gain=R/L
  "R/L " : Gain  Gain=R/L
  Sum2 : Sum  Inputs=|+-
  Sum5 : Sum  Inputs=|+-
  Ialpha^ : Outport
  Ibeta^ : Outport  Port=2
  wires:
  Ibeta*/1 -> " 1/L "/1
  Ialfa*/1 -> "1/L "/1
  Ialfa/1 -> Sum2/2
  Ibeta/1 -> Sum5/2
  Sum5/1 -> Ibeta^/1
  Integrator1/1 -> "R/L "/1, Sum5/1
  Ubeta/1 -> " 1/L"/1
  1/L/1 -> " "/1
  Sum2/1 -> Ialpha^/1
  " 1/L"/1 -> "   "/1
  " "/1 -> Integrator/1
  Ualfa/1 -> 1/L/1
  " 1/L "/1 -> "   "/3
  Integrator/1 -> R/L/1, Sum2/1
  "R/L "/1 -> "   "/2
  "1/L "/1 -> " "/3
  "   "/1 -> Integrator1/1
  R/L/1 -> " "/2
